simulink model "AdecuacionEMG2"  (Simulink 6.6)
settings: Solver=ode45  StartTime=0.0  StopTime=100  RelTol=1e-3
undefined symbols (not defined in the file or in its folder): get
libraries: dspsnks4 x4, dsparch4 x2, dspwin32 x2, dspbuff3 x1
settings Model: Creator=F565la07hrfjn  LastModifiedBy=F565la07hrfjn
settings DebuggingCC: SolverPrmCheckMsg=none

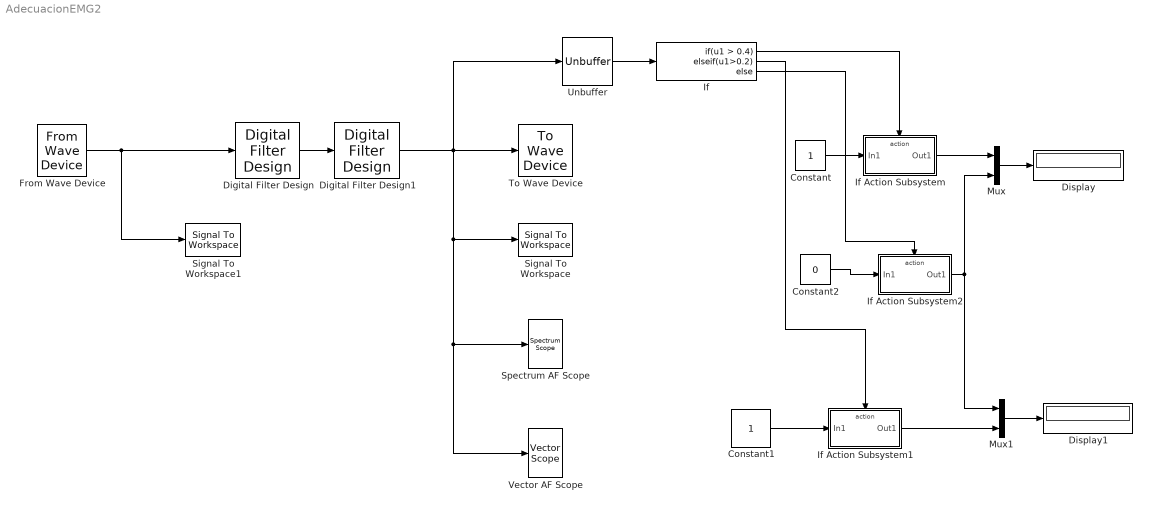
== system AdecuacionEMG2 ==
  Constant : Constant
  Constant1 : Constant
  Constant2 : Constant  Value=0
  Digital Filter Design : dsparch4/Digital Filter Design  SystemSampleTime=-1  mwdsp_browser_bugfix_var=off
  Digital Filter Design1 : dsparch4/Digital Filter Design  SystemSampleTime=-1  mwdsp_browser_bugfix_var=off
  Display : Display
  Display1 : Display
  From Wave Device : dspwin32/From Wave Device  SampleRate=44100  UserRate=16000  SampleWidth=8  Stereo=off  SamplesPerFrame=512  QueueDuration=3  useDefaultDevice=on  userDeviceID=Micrófono (Conexant High Defini  dType=double
  If : If  IfExpression=u1 > 0.4  ElseIfExpressions=u1>0.2  ZeroCross=off
  If Action Subsystem : Subsystem  TreatAsAtomicUnit=on
  If Action Subsystem1 : Subsystem  TreatAsAtomicUnit=on
  If Action Subsystem2 : Subsystem  TreatAsAtomicUnit=on
  Mux : Mux  Inputs=2
  Mux1 : Mux  Inputs=2
  Signal To Workspace : dspsnks4/Signal To Workspace  SystemSampleTime=-1  VariableName=AF  FrameMode=Concatenate frames (2-D array)
      settings: FixptAsFi=off
  Signal To Workspace1 : dspsnks4/Signal To Workspace  SystemSampleTime=-1  VariableName=BF  FrameMode=Concatenate frames (2-D array)
      settings: FixptAsFi=off
  Spectrum AF Scope : dspsnks4/Spectrum Scope  DialogController=dspdialog.SpectrumScope  DialogControllerArgs=DataTag2  SystemSampleTime=-1  ScopeProperties=on  Domain=Frequency  HorizSpan=1  UseBuffer=off  BufferSize=128  Overlap=64  inpFftLenInherit=off  FFTlength=128  numAvg=2  DisplayProperties=off  AxisGrid=on  Memory=off  FrameNumber=on  AxisLegend=off  AxisZoom=off  OpenScopeAtSimStart=on  OpenScopeImmediately=off  FigPos=get(0,'defaultfigureposition')  AxisProperties=off  XUnits=Hertz  XRange=[0...Fs/2]  InheritXIncr=on  XIncr=1.0  XLabel=Samples  XLimit=Auto  YUnits=dB  XMax=1  XMin=0  YLabel=Magnitude-squared, dB  LineProperties=off  wintypeSpecScope=Hann  RsSpecScope=50  betaSpecScope=5  winsampSpecScope=Periodic
      settings: YMin=-30  YMax=10
  To Wave Device : dspwin32/To Wave Device  bufDuration=2  determineBufSize=on  userIntBufSize=256  initDelay=0.1  useDefaultDevice=on  userDeviceID=Altavoz y auricular interno (Co  enable24Bit=off
  Unbuffer : dspbuff3/Unbuffer  ic=0
  Vector AF Scope : dspsnks4/Vector Scope  DialogController=dspdialog.VectorScope  DialogControllerArgs=DataTag3  ScopeProperties=on  Domain=Time  HorizSpan=1  DisplayProperties=off  AxisGrid=on  Memory=off  FrameNumber=on  AxisLegend=off  AxisZoom=off  OpenScopeAtSimStart=on  OpenScopeImmediately=off  FigPos=get(0,'defaultfigureposition')  AxisProperties=off  XUnits=Hertz  XRange=[0...Fs/2]  InheritXIncr=on  XIncr=1  XLabel=Time  XLimit=User-defined  XMin=0  XMax=10  XStart=0  YUnits=dB  YLabel=Amplitude  LineProperties=off
      settings: YMin=-1  YMax=1
  wires:
  Digital Filter Design/1 -> Digital Filter Design1/1
  Digital Filter Design1/1 -> Signal To Workspace/1, Spectrum AF Scope/1, Vector AF Scope/1, Unbuffer/1, To Wave Device/1
  From Wave Device/1 -> Digital Filter Design/1, Signal To Workspace1/1
  Unbuffer/1 -> If/1
  If/1 -> If Action Subsystem/Action
  Constant/1 -> If Action Subsystem/1(In1)
  If/2 -> If Action Subsystem1/Action
  Constant1/1 -> If Action Subsystem1/1(In1)
  If/3 -> If Action Subsystem2/Action
  Constant2/1 -> If Action Subsystem2/1(In1)
  If Action Subsystem/1(Out1) -> Mux/1
  Mux/1 -> Display/1
  If Action Subsystem2/1(Out1) -> Mux/2, Mux1/1
  If Action Subsystem1/1(Out1) -> Mux1/2
  Mux1/1 -> Display1/1

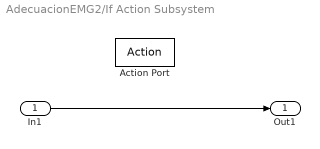
== system AdecuacionEMG2/If Action Subsystem ==
  In1 : Inport
  Action Port : ActionPort  InitializeStates=reset  ActionType=then
  Out1 : Outport
  wires:
  In1/1 -> Out1/1

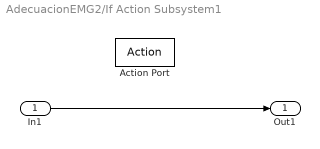
== system AdecuacionEMG2/If Action Subsystem1 ==
  In1 : Inport
  Action Port : ActionPort  InitializeStates=reset  ActionType=elseif
  Out1 : Outport
  wires:
  In1/1 -> Out1/1

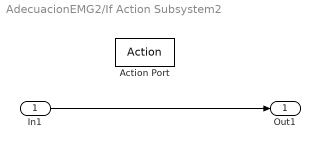
== system AdecuacionEMG2/If Action Subsystem2 ==
  In1 : Inport
  Action Port : ActionPort  InitializeStates=reset  ActionType=else
  Out1 : Outport
  wires:
  In1/1 -> Out1/1
